simulink model "electrolyser_test"  (R2022a)
settings: Solver=VariableStepAuto  StartTime=0.0  StopTime=10.0  RelTol=1e-3
model workspace: external: MATLAB File parameters_straight.m (data not in the file)
undefined symbols (not defined in the file or in its folder): const
libraries: fl_lib x8, SimscapeFluids_lib x3
(part 2 of 2)

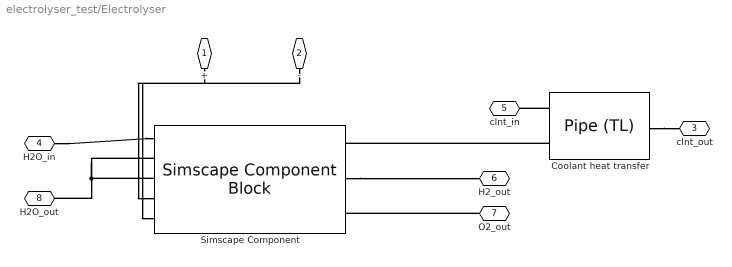
== system electrolyser_test/Electrolyser ==
  Coolant heat transfer : SimscapeFluids_lib/Thermal Liquid/Pipes & Fittings/Pipe (TL)  dynamic_compressibility=simscape.enum.onoff.off  inertia=simscape.enum.onoff.off  num_segments=pemel.N_clt  pipe_length=pemel.L_clt m  area=0.01 m^2  wall_spec=fluids.thermal_liquid.pipes_fittings.enum.wall_spec.rigid  Dh=0.1128 m  wall_compliance=1.2e-6 m/MPa  wall_time_constant=0.01 s  elevation_spec=foundation.enum.constant_variable.constant  elevation_gain=0 m  g=9.81 m/s^2  pressure_loss_spec=fluids.thermal_liquid.pipes_fittings.enum.PressureLossSpec.Haaland  local_pressure_loss_spec=fluids.thermal_liquid.pipes_fittings.enum.LocalLossSpec.AggregateLength  length_add=1 m  loss_coefficient=0.1  roughness=15e-6 m  Re_friction_TLU=[400, 1000, 1500, 3000, 4000, 6000, 10000, 20000, 40000, 60000, 100000, 100000000]  friction_factor_TLU=[.264, .112, .071, .0417, .0387, .0268, .025, .0232, .0226, .022, .0214, .0214]  shape_factor=64  Re_lam=2000  Re_tur=4000  mdot_nominal=[.1, 1] kg/s  p_diff_nominal=[.001, .01] MPa  mdot_threshold=1e-6 kg/s  heat_transfer_spec=fluids.thermal_liquid.pipes_fittings.enum.HeatTransferSpec.Gnielinski  mdot_nominal_heat=[.1, 1] kg/s  T_in_nominal=[293.15, 293.15] K  T_out_nominal=[300, 300] K  p_in_nominal_heat=[.101325, .101325] MPa  T_wall_nominal=[303.15, 303.15] K  a_coeff=0.023  b_Re_power=0.8  c_Pr_power=0.4  Nu_lam=3.66  Re_Colburn_TLU=[100, 150, 1000]  Colburn_factor_TLU=[.019, .013, .002]  Re_Nu_TLU=[100, 150, 1000]  Pr_Nu_TLU=[1, 10]  Nu_TLU=[3.72, 4.21; 3.75, 4.44; 4.21, 7.15]  T0_vec=293.15 K  p0_vec=0.101325 MPa  mdot0=0.1 kg/s
      settings: SourceProductBaseCode=SH
  Simscape Component : SimscapeComponentBlock  SourceFile=electrolyser  ComponentPath=electrolyser  ComponentVariants="[\"electrolyser\"]"  ComponentVariantNames="[\"electrolyser\"]"  ClassName=electrolyser  SchemaVersion=1  T_ref=293.15 K  p_ref=101325 Pa  HHV_h2=1.419E8 J/kg  rho_h2=0.082 kg/m^3  rho_o2=1.31 kg/m^3  rho_h2o=1000 kg/m^3  M_h2=0.0020158 kg/mol  M_o2=0.0319988 kg/mol  M_h2o=0.0180152 kg/mol  N_cel=30  A_cel=0.1 m^2  vol_ca=0.1 m^3  vol_an=0.005 m^3  A_mem=0.1 m^2  thk_mem=0.178 mm  rho_mem=0.001 kg/m^3  V_stk_i=[1.2 : 0.5 : 3] V  J_stk_i=[1.2 : 0.5 : 3] A/m^2  m_bp=1 kg  cp_bp=100 J/kg/K  cp_mem=1 J/(K*kg)  mdot_h2o_in_specify=off  mdot_h2o_in_priority=None  mdot_h2o_in=0 kg/s  mdot_h2o_in_nominal_specify=off  mdot_h2o_in_nominal_unit=kg/s  mdot_h2o_in_nominal_value=1  mdot_h2o_out_an_specify=off  mdot_h2o_out_an_priority=None  mdot_h2o_out_an=0 kg/s  mdot_h2o_out_an_nominal_specify=off  mdot_h2o_out_an_nominal_unit=kg/s  mdot_h2o_out_an_nominal_value=1  mdot_h2o_out_ca_specify=off  mdot_h2o_out_ca_priority=None  mdot_h2o_out_ca=0 kg/s  mdot_h2o_out_ca_nominal_specify=off  mdot_h2o_out_ca_nominal_unit=kg/s  mdot_h2o_out_ca_nominal_value=1  mdot_o2_out_specify=off  mdot_o2_out_priority=None  mdot_o2_out=0 kg/s  mdot_o2_out_nominal_specify=off  mdot_o2_out_nominal_unit=kg/s  mdot_o2_out_nominal_value=1  mdot_h2_out_specify=off  mdot_h2_out_priority=None  mdot_h2_out=0 kg/s  mdot_h2_out_nominal_specify=off  mdot_h2_out_nominal_unit=kg/s  mdot_h2_out_nominal_value=1  Phi_h2o_in_specify=off  Phi_h2o_in_priority=None  Phi_h2o_in=0 W  Phi_h2o_in_nominal_specify=off  Phi_h2o_in_nominal_unit=W  Phi_h2o_in_nominal_value=1  Phi_h2o_out_an_specify=off  Phi_h2o_out_an_priority=None  Phi_h2o_out_an=0 W  Phi_h2o_out_an_nominal_specify=off  Phi_h2o_out_an_nominal_unit=W  Phi_h2o_out_an_nominal_value=1  Phi_h2o_out_ca_specify=off  Phi_h2o_out_ca_priority=None  Phi_h2o_out_ca=0 W  Phi_h2o_out_ca_nominal_specify=off  Phi_h2o_out_ca_nominal_unit=W  Phi_h2o_out_ca_nominal_value=1  Phi_o2_out_specify=off  Phi_o2_out_priority=None  Phi_o2_out=0 W  Phi_o2_out_nominal_specify=off  Phi_o2_out_nominal_unit=W  Phi_o2_out_nominal_value=1  Phi_h2_out_specify=off  Phi_h2_out_priority=None  Phi_h2_out=0 W  Phi_h2_out_nominal_specify=off  Phi_h2_out_nominal_unit=W  Phi_h2_out_nominal_value=1  I_specify=off  I_priority=None  I=0 A  I_nominal_specify=off  I_nominal_unit=A  I_nominal_value=1  T_stk_specify=off  T_stk_priority=None  T_stk=293.15 K  T_stk_nominal_specify=off  T_stk_nominal_unit=K  T_stk_nominal_value=1  mass_h2o_an_specify=off  mass_h2o_an_priority=None  mass_h2o_an=0 kg  mass_h2o_an_nominal_specify=off  mass_h2o_an_nominal_unit=kg  mass_h2o_an_nominal_value=1  mass_h2o_ca_specify=off  mass_h2o_ca_priority=None  mass_h2o_ca=0 kg  mass_h2o_ca_nominal_specify=off  mass_h2o_ca_nominal_unit=kg  mass_h2o_ca_nominal_value=1  mass_o2_specify=off  mass_o2_priority=None  mass_o2=0 kg  mass_o2_nominal_specify=off  mass_o2_nominal_unit=kg  mass_o2_nominal_value=1  mass_h2_specify=off  mass_h2_priority=None  mass_h2=0 kg  mass_h2_nominal_specify=off  mass_h2_nominal_unit=kg  mass_h2_nominal_value=1  p_o2_specify=off  p_o2_priority=None  p_o2=1 atm  p_o2_nominal_specify=off  p_o2_nominal_unit=atm  p_o2_nominal_value=1  p_h2_specify=off  p_h2_priority=None  p_h2=1 atm  p_h2_nominal_specify=off  p_h2_nominal_unit=atm  p_h2_nominal_value=1  p_h2o_an_specify=off  p_h2o_an_priority=None  p_h2o_an=1 atm  p_h2o_an_nominal_specify=off  p_h2o_an_nominal_unit=atm  p_h2o_an_nominal_value=1  p_h2o_ca_specify=off  p_h2o_ca_priority=None  p_h2o_ca=1 atm  p_h2o_ca_nominal_specify=off  p_h2o_ca_nominal_unit=atm  p_h2o_ca_nominal_value=1  Qdot_clnt_specify=off  Qdot_clnt_priority=None  Qdot_clnt=0 W  Qdot_clnt_nominal_specify=off  Qdot_clnt_nominal_unit=W  Qdot_clnt_nominal_value=1
      settings: CopyFcn=simscape.engine.sli.internal.componentblockcallback(gcbh,'COPY')  PreCopyFcn=simscape.engine.sli.internal.componentblockcallback(gcbh,'PRECOPY')  PreDeleteFcn=simscape.engine.sli.internal.componentblockcallback(gcbh,'PREDELETE')  InternalSimscapePortConfiguration="{\"Bottom\":[],\"Left\":[{\"id\":\"h2o_in\",\"label\":\"H2O_in\",\"type\":\"foundation.thermal_liquid.thermal_liquid\"},{\"id\":\"h2o_out_an\",\"label\":\"H2O_out_an\",\"type\":\"foundation.thermal_liquid.thermal_liquid\"},{\"id\":\"h2o_out_ca\",\"label\":\"H2O_out_ca\",\"type\":\"foundation.thermal_liquid.thermal_liquid\"}],\"Right\":[{\"id\":\"clnt_Qout\",\"label\":\"Qdot_clnt\",\"type\":\"foundation.thermal.thermal\"},{\"id\":\"h2_out\",\"label\":\"H2_out\",\"type\":\"foundation.gas.gas\"},{\"id\":\"o2_out\",\"label\":\"O2_out\",\"type\":\"foundation.gas.gas\"}],\"Top\":[{\"id\":\"elec_pos\",\"label\":\"+\",\"type\":\"foundation.electrical.electrical\"},{\"id\":\"elec_neg\",\"label\":\"\\u001a\",\"type\":\"foundation.electrical.electrical\"}]}"
      mask Type: Two-port dynamic two-phase fluid component
  + : PMIOPort  Side=Left
  - : PMIOPort  Port=2  Side=Left
  clnt_out : PMIOPort  Port=3  Side=Left
  H2O_in : PMIOPort  Port=4  Side=Left
  clnt_in : PMIOPort  Port=5  Side=Right
  H2_out : PMIOPort  Port=6  Side=Right
  O2_out : PMIOPort  Port=7  Side=Right
  H2O_out : PMIOPort  Port=8  Side=Right
  connections:
  Simscape Component/RConn2 -- H2_out/RConn1
  -/RConn1 -- Simscape Component/LConn5
  O2_out/RConn1 -- Simscape Component/RConn3
  +/RConn1 -- Simscape Component/LConn4
  Simscape Component/LConn2 -- Simscape Component/LConn3 -- H2O_out/RConn1
  H2O_in/RConn1 -- Simscape Component/LConn1
  Coolant heat transfer/LConn2 -- Simscape Component/RConn1
  Coolant heat transfer/RConn1 -- clnt_out/RConn1
  Coolant heat transfer/LConn1 -- clnt_in/RConn1
